simulink model "lab6_report_model"  (R2014a)
settings: Solver=ode45  StartTime=0.0  StopTime=3.0  MaxStep=.001  RelTol=1e-3
values from neighbouring files (symbols this model uses):
  K = 18.246    [lab6reportcode.m]
  K_amp = 2.4    [lab6reportcode.m]
  K_c = 3.1    [lab6reportcode.m]
  K_pot = 10/(2*pi)    (= 1.59154943092)    [lab6reportcode.m]
  t_m = 4.131    [lab6reportcode.m]    (also in prelab6.m = 0.2)
  t_p = .0045    (= 0.0045)    [lab6reportcode.m]    (also in prelab6.m = 0.0108695652174)
  t_z = .034    (= 0.034)    [lab6reportcode.m]    (also in prelab6.m = 0.434782608696)
settings Model: Creator=nandi2  LastModifiedBy=Matthew
settings DataIOCC: LimitDataPoints=off

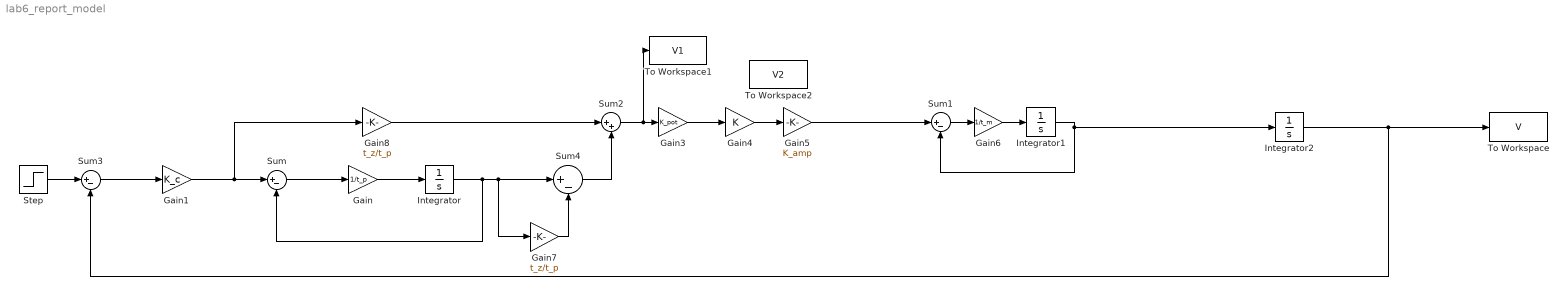
== system lab6_report_model ==
  Gain : Gain  Gain=1/t_p
  Gain1 : Gain  Gain=K_c
  Gain3 : Gain  Gain=K_pot
  Gain4 : Gain  Gain=K
  Gain5 : Gain  Gain=K_amp
  Gain6 : Gain  Gain=1/t_m
  Gain7 : Gain  Gain=t_z/t_p
  Gain8 : Gain  Gain=t_z/t_p
  Integrator : Integrator
  Integrator1 : Integrator
  Integrator2 : Integrator
  Step : Step  Time=0  SampleTime=0
  Sum{,1,3..4} (4 alike) : Sum  Inputs=|+-
  Sum2 : Sum  Inputs=|++
  To Workspace : ToWorkspace  VariableName=V  SampleTime=-1
  To Workspace1 : ToWorkspace  VariableName=V1  SampleTime=-1
  To Workspace2 : ToWorkspace  VariableName=V2  SampleTime=-1
  wires:
  Gain1/1 -> Gain8/1, Sum/1
  Sum/1 -> Gain/1
  Gain8/1 -> Sum2/1
  Gain/1 -> Integrator/1
  Sum3/1 -> Gain1/1
  Integrator/1 -> Gain7/1, Sum4/1, Sum/2
  Gain3/1 -> Gain4/1
  Gain4/1 -> Gain5/1
  Gain5/1 -> Sum1/1
  Sum1/1 -> Gain6/1
  Gain6/1 -> Integrator1/1
  Step/1 -> Sum3/1
  Sum2/1 -> Gain3/1, To Workspace1/1
  Sum4/1 -> Sum2/2
  Gain7/1 -> Sum4/2
  Integrator1/1 -> Integrator2/1, Sum1/2
  Integrator2/1 -> Sum3/2, To Workspace/1
